simulink model "Converting_Kg_to_Pounds"  (R2021a)
settings: Solver=VariableStepAuto  StartTime=0.0  StopTime=10.0  RelTol=1e-3
settings Model: Creator=HP  LastModifiedBy=HP

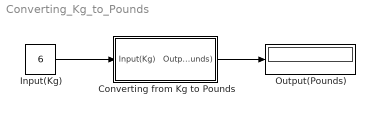
== system Converting_Kg_to_Pounds ==
  Converting from Kg to Pounds : Subsystem
  Input(Kg) : Constant  Value=6
  Output(Pounds) : Display
  wires:
  Converting from Kg to Pounds/1(Output(pounds)) -> Output(Pounds)/1
  Input(Kg)/1 -> Converting from Kg to Pounds/1(Input(Kg))

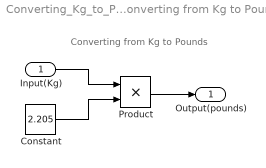
== system Converting_Kg_to_Pounds/Converting from Kg to Pounds ==
  note: Converting from Kg to Pounds
  Input(Kg) : Inport
  Constant : Constant  Value=2.205
  Product : Product
  Output(pounds) : Outport
  wires:
  Product/1 -> Output(pounds)/1
  Input(Kg)/1 -> Product/1
  Constant/1 -> Product/2
